simulink model "mind"  (R2022b)
settings: Solver=FixedStepAuto  StartTime=0.0  StopTime=inf  RelTol=1e-3  EnableMultiTasking=on
undefined symbols (not defined in the file or in its folder): DiscIntNeverNeededParam, GRM_discrete, HinfDiscrete, K, Observer, PID, Red
libraries: arduinolib x5, simulink x1, slpidlib x1
settings Model: SimulationMode=external  ExtModeTrigDuration=2  Creator=amoralesma  LastModifiedBy=amoralesma
settings DataIOCC: ReturnWorkspaceOutputs=off
settings OptimizationCC: EnhancedBackFolding=on  PassReuseOutputArgsAs=Individual arguments  ZeroExternalMemoryAtStartup=off  ZeroInternalMemoryAtStartup=off  MaxStackSize=64  OptimizeBlockOrder=speed  DifferentSizesBufferReuse=on  OptimizationCustomize=off  EfficientTunableParamExpr=on
settings DebuggingCC: ParameterTunabilityLossMsg=error
settings HardwareCC: ProdBitPerInt=16  ProdBitPerPointer=16  ProdBitPerSizeT=16  ProdBitPerPtrDiffT=16  ProdLargestAtomicFloat=None  ProdWordSize=8  ProdHWDeviceType=Atmel->AVR  UseEmbeddedCoderFeatures=off  UseSimulinkCoderFeatures=off
settings SFSimCC: MATLABDynamicMemAlloc=off
settings RTWCC: Description=Embedded Coder  SystemTargetFile=ert.tlc  HardwareBoard=Arduino Mega 2560  TemplateMakefile=ert_default_tmf  RTWVerbose=off  Toolchain=Arduino AVR  BuildConfiguration=Faster Runs
settings CodeAppCC: ForceParamTrailComments=on  OperatorAnnotations=on  SimulinkDataObjDesc=on  SFDataObjDesc=on  MangleLength=10  InsertBlockDesc=on
settings ERTTargetCC: SupportContinuousTime=on  SupportNonInlinedSFcns=on  SupportVariableSizeSignals=on  ExtMode=on  ExtModeTransport=3  ExtModeStaticAlloc=on  ExtModeAutomaticAllocSize=off  ExtModeStaticAllocSize=2048  ExtModeMexFile=ext_xcp  ExtModeMexArgs=0 '/dev/cu.usbserial-14110' 115200  ExtModeIntrfLevel=Level2 - Open  ERTSrcFileBannerTemplate=codertarget_code_template.cgt  ERTHdrFileBannerTemplate=codertarget_code_template.cgt  ERTDataSrcFileTemplate=codertarget_code_template.cgt  ERTDataHdrFileTemplate=codertarget_code_template.cgt

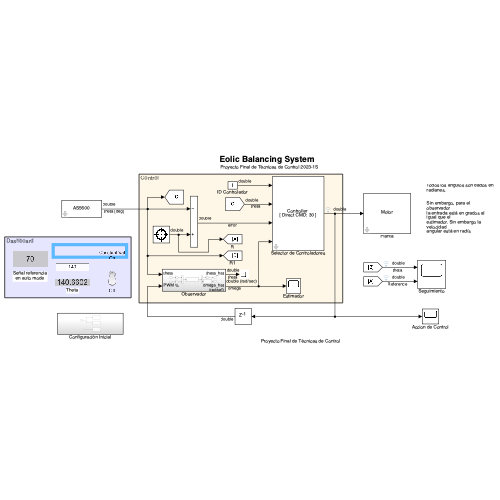
[thumbnail: Simulink's stored preview of the top-level diagram]
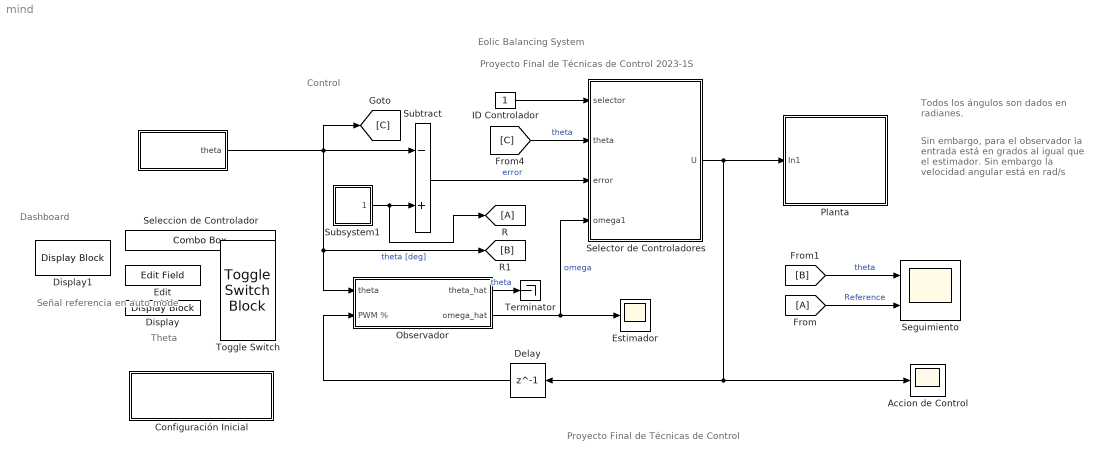
== system mind ==
  note: Señal referencia
      | en auto mode
  note: Dashboard
  note: Todos los ángulos son dados en
      | radianes.
  note: Control
  note: Eolic Balancing System
  note: Proyecto Final de Técnicas de Control 2023-1S
  note: Sin embargo, para el observador
      | la entrada está en grados al igual que el
      | estimador. Sin embargo la velocidad
      | angular está en rad/s
  note: Proyecto Final de Técnicas de Control
  note: Theta
  " " : Subsystem
      mask Display: disp('AS5600');
  Accion de Control : Scope
  Configuración Inicial : Subsystem
  Delay : Delay  DelayLength=1
  Display : DisplayBlock  LabelPosition=Hide  Transparency=1
  Display1 : DisplayBlock  LabelPosition=Hide  Transparency=1
  Edit : EditField  LabelPosition=Hide  ShowInitialText=on  Alignment=Center
  Estimador : Scope
  From : From
  ID Controlador : Constant  SampleTime=0.0025
  Observador : Subsystem
  Planta : Subsystem
      mask Display: disp('Motor');
  R : Goto
  Seguimiento : Scope  NumInputPorts=2
  Seleccion de Controlador : ComboBox  LabelPosition=Hide  SelectedLabel=PID + Red
      settings: Values={{'PID + Red', 'SMC', 'H-infinito', 'SMC + tanh', 'SMC + equivalente', 'MRAC', 'LQR', 'LQG'}, [1 2 3 4 5 6 7 8]}
  Selector de Controladores : Subsystem  mask{accionControlDirecta=30}
      mask prompts: accionControlDirecta "Accion de Control Directa"
      mask DialogControl DescTextVar Prompt: Selector de controladores. Varía el controlador en función del a entrada ID
      mask Display: disp("Controller \n[ Direct CMD: " + get_param(gcb, "accionControlDirecta") + " ]");
  Subsystem1 : Subsystem
      mask Display: image('/Users/amoralesma/Documents/UN/TdC/eolic-balancing-cs/implementacion/assets/target_icon.png'); % Use "Edit Image" on toolstrip to change.
  Subtract : Sum  Inputs=-+
  Terminator : Terminator
  Toggle Switch : ToggleSwitchBlock
      settings: Values={{'Off', 'On'}, [0 1]}
  wires:
  " "/1(theta) -> [C], Subtract/1, [B], Observador/1(theta)  "theta [deg]"
  Subtract/1 -> Selector de Controladores/3(error)  "error"
  Selector de Controladores/1(U) -> Delay/1, Accion de Control/1, Planta/1(In1)
  ID Controlador/1 -> Selector de Controladores/1(selector)
  Observador/2(omega_hat) -> Selector de Controladores/4(omega1), Estimador/1  "omega"
  Delay/1 -> Observador/2(PWM %)
  From/1 -> Seguimiento/2  "Reference"
  [B] -> Seguimiento/1  "theta"
  Observador/1(theta_hat) -> Terminator/1  "theta"
  [C] -> Selector de Controladores/2(theta)  "theta"
  Subsystem1/1(Out2) -> R/1, Subtract/2

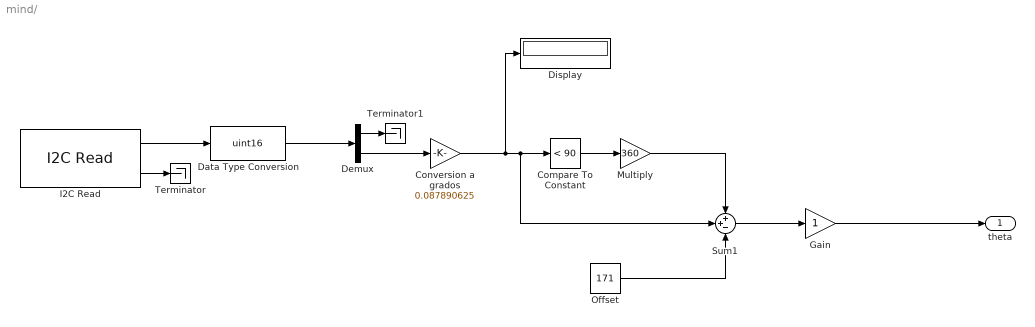
== system mind/  ==
  Compare To Constant : simulink/Logic and Bit Operations/Compare To Constant  relop=<  const=90  OutDataTypeStr=uint8
  Conversion a grados : Gain  Gain=0.087890625
  Data Type Conversion : DataTypeConversion  OutDataTypeStr=uint16  SaturateOnIntegerOverflow=off  RndMeth=Floor
  Demux : Demux  Outputs=2
  Display : Display
  Gain : Gain
  I2C Read : arduinolib/I2C Read  I2CModule=0  Mode=Master  SlaveAddress=0x36  SlaveByteOrder=BigEndian  Direction=Receiver  RegisterAddressMode=on  RegisterAddress=0x0C  SlaveDataType=uint16  DataLength=2  NoAck=off  RepeatedStart=off  OutputStatus=on  blockPlatform=ARDUINO  SampleTime=-1
  Multiply : Gain  Gain=360
  Offset : Constant  Value=171
  Sum1 : Sum  Inputs=++-
  Terminator : Terminator
  Terminator1 : Terminator
  theta : Outport
  wires:
  Demux/2 -> Conversion a grados/1
  Data Type Conversion/1 -> Demux/1
  Offset/1 -> Sum1/3
  I2C Read/1 -> Data Type Conversion/1
  Multiply/1 -> Sum1/1
  Conversion a grados/1 -> Display/1, Compare To Constant/1, Sum1/2
  Compare To Constant/1 -> Multiply/1
  I2C Read/2 -> Terminator/1
  Sum1/1 -> Gain/1
  Demux/1 -> Terminator1/1
  Gain/1 -> theta/1

== system mind/Configuración Inicial ==
  Constant : Constant
  Constant1 : Constant  Value=0
  EN1 : arduinolib/Digital Output  pinNumber=11  Direction=output  blockPlatform=arduino
  EN2 : arduinolib/Digital Output  pinNumber=12  Direction=output  blockPlatform=arduino
  IN3 : arduinolib/Digital Output  pinNumber=6  Direction=output  blockPlatform=arduino
  wires:
  Constant/1 -> EN2/1, EN1/1
  Constant1/1 -> IN3/1

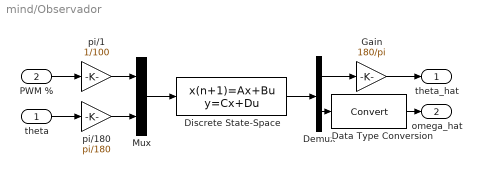
== system mind/Observador ==
  theta : Inport
  PWM % : Inport  Port=2
  Data Type Conversion : DataTypeConversion  SaturateOnIntegerOverflow=off  RndMeth=Floor
  Demux : Demux  Outputs=2
  Discrete State-Space : DiscreteStateSpace  A=Observer.A  B=Observer.B  C=Observer.C  D=Observer.D  SampleTime=-1
  Gain : Gain  Gain=180/pi
  Mux : Mux  Inputs=2
  pi/1 : Gain  Gain=1/100  OutDataTypeStr=Inherit: Same as input
  pi/180 : Gain  Gain=pi/180
  theta_hat : Outport
  omega_hat : Outport  Port=2  Unit=rad/sec
  wires:
  Mux/1 -> Discrete State-Space/1
  theta/1 -> pi/180/1
  Discrete State-Space/1 -> Demux/1
  pi/180/1 -> Mux/2
  PWM %/1 -> pi/1/1
  pi/1/1 -> Mux/1
  Gain/1 -> theta_hat/1
  Demux/1 -> Gain/1
  Demux/2 -> Data Type Conversion/1
  Data Type Conversion/1 -> omega_hat/1

== system mind/Planta ==
  In1 : Inport
  Gain1 : Gain  Gain=255/100
  PWM : arduinolib/PWM  pinNumber=7  frequencyType=Default  desiredFrequency=490.2  achievableFrequency=490.2
  wires:
  In1/1 -> Gain1/1
  Gain1/1 -> PWM/1

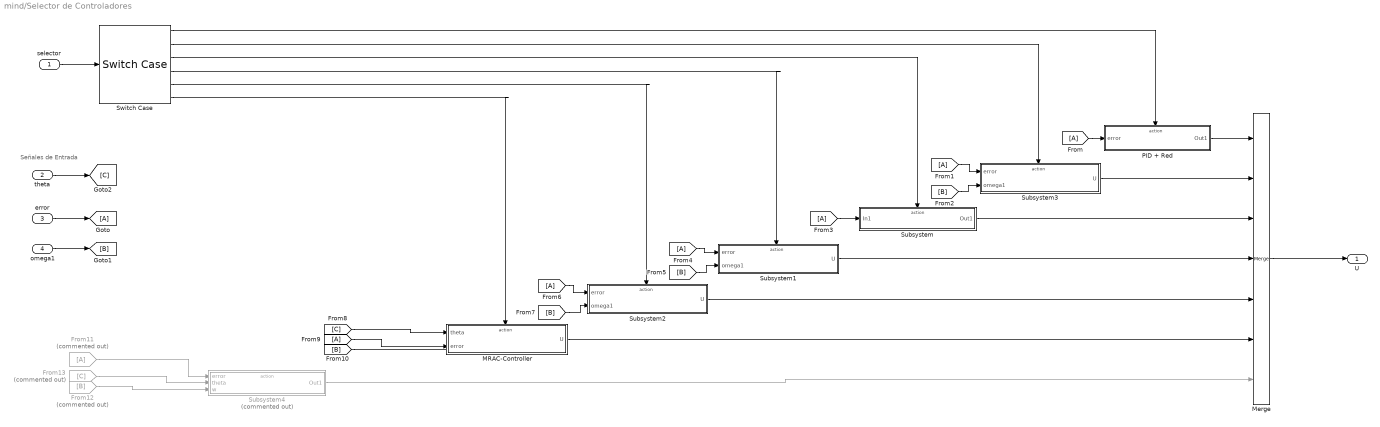
== system mind/Selector de Controladores ==
  note: Señales de Entrada
  selector : Inport
  theta : Inport  Port=2
  error : Inport  Port=3
  omega1 : Inport  Port=4
  From{,1,3..4,6,9} (6 alike) : From
  From11 : From  Commented=on
  From12 : From  Commented=on  GotoTag=B
  From13 : From  Commented=on  GotoTag=C
  Goto : Goto
  MRAC-Controller : Subsystem  mask{directCMD=accionControlDirecta, gx=7, gr=0.3}
      mask prompts: directCMD "CMD"; gx "Gamma X"; gr "Gamma R"
      mask DialogControl Control2 Prompt: Propiedades de MRAC
      mask Display:
      | disp('MRAC');
      | 
      | port_label('input', 1, 'theta');
      | port_label('input', 2, 'error');
      | port_label('input', 3, 'omega');
      | 
      | port_label('output', 1, 'u');
  Merge : Merge  Inputs=7
  PID + Red : Subsystem  mask{directCMD=accionControlDirecta}
      mask prompts: directCMD "Accion de control directa"
      mask Display: disp('PID');
  Subsystem : Subsystem
      mask Display: disp('H-inf');
  Subsystem1 : Subsystem
      mask Display:
      | disp('SMC + tanh');
      | 
      | port_label('input', 1, 'error');
      | port_label('input', 2, 'omega (x2)');
      | 
      | port_label('output', 1, 'u');
  Subsystem2 : Subsystem
      mask Display:
      | disp('SMC + eq');
      | 
      | port_label('input', 1, 'error');
      | port_label('input', 2, 'omega (x2)');
      | 
      | port_label('output', 1, 'u');
  Subsystem3 : Subsystem
      mask Display:
      | disp('SMC');
      | 
      | port_label('input', 1, 'error');
      | port_label('input', 2, 'omega (x2)');
      | 
      | port_label('output', 1, 'u');
  Subsystem4 : Subsystem  Commented=on
      mask Display: disp('LQR');
  Switch Case : SwitchCase  CaseConditions={1, 2,3, 4, 5,6,}  ShowDefaultCase=off
  U : Outport
  wires:
  Switch Case/1 -> PID + Red/Action
  Switch Case/2 -> Subsystem3/Action
  error/1 -> Goto/1
  omega1/1 -> [B]
  From/1 -> PID + Red/1(error)
  From1/1 -> Subsystem3/1(error)
  [B] -> Subsystem3/2(omega1)
  PID + Red/1(Out1) -> Merge/1
  Subsystem3/1(U) -> Merge/2
  selector/1 -> Switch Case/1
  From3/1 -> Subsystem/1(In1)
  Subsystem/1(Out1) -> Merge/3
  Switch Case/3 -> Subsystem/Action
  Merge/1 -> U/1
  Switch Case/4 -> Subsystem1/Action
  Switch Case/5 -> Subsystem2/Action
  From4/1 -> Subsystem1/1(error)
  [B] -> Subsystem1/2(omega1)
  From6/1 -> Subsystem2/1(error)
  [B] -> Subsystem2/2(omega1)
  Subsystem1/1(U) -> Merge/4
  Subsystem2/1(U) -> Merge/5
  Switch Case/6 -> MRAC-Controller/Action
  theta/1 -> [C]
  [C] -> MRAC-Controller/1(theta)
  From9/1 -> MRAC-Controller/2(error)
  MRAC-Controller/1(U) -> Merge/6
  [B] -> ?
  Subsystem4/1(Out1) -> Merge/7
  From13/1 -> Subsystem4/2(theta)
  From12/1 -> Subsystem4/3(w)
  From11/1 -> Subsystem4/1(error)

== system mind/Subsystem1 ==
  Constant : Constant  Value=0
  Ref : Constant  Value=140
  Subsystem : Subsystem
  Switch : Switch  Criteria=u2 ~= 0  SaturateOnIntegerOverflow=off  InputSameDT=off
  Out2 : Outport
  wires:
  Switch/1 -> Out2/1
  Constant/1 -> Switch/2
  Subsystem/1(Out1) -> Switch/1
  Ref/1 -> Switch/3

== system mind/Selector de Controladores/MRAC-Controller ==
  theta : Inport
  error : Inport  Port=2
  Action Port : ActionPort  ActionPortLabel=case [ 6 ]:
  Gain : Gain  Gain=pi/180
  Gain1 : Gain  Gain=pi/180
  MRAC : Subsystem
  U : Outport
  wires:
  theta/1 -> Gain/1
  error/1 -> Gain1/1
  Gain1/1 -> MRAC/2(error)
  MRAC/1(U) -> U/1
  Gain/1 -> MRAC/1(theta)

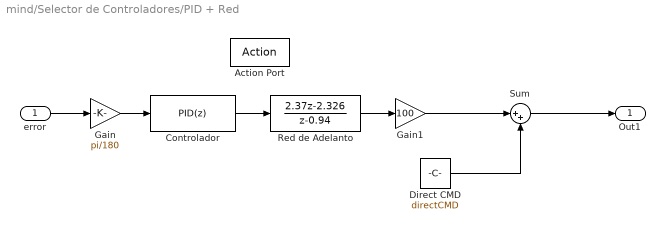
== system mind/Selector de Controladores/PID + Red ==
  error : Inport
  Action Port : ActionPort  ActionPortLabel=case [ 1 ]:
  Controlador : slpidlib/PID Controller  Controller=PID  Form=Parallel  TimeDomain=Discrete-time  UseExternalTs=off  SampleTime=0.0025  IntegratorMethod=Forward Euler  FilterMethod=Forward Euler  ControllerParametersSource=internal  P=0.4  I=0.65  UseKiTs=off  D=0.018  N=100  UseFilter=off  TunerSelectOption=Transfer Function Based (PID Tuner App)  InitialConditionSource=internal  InitialConditionForIntegrator=0  InitialConditionForFilter=0  DifferentiatorICPrevScaledInput=0  ExternalReset=none  TrackingMode=off  Kt=1  LimitOutput=on  SatLimitsSource=internal  UpperSaturationLimit=70  LowerSaturationLimit=-30  LinearizeAsGain=off  AntiWindupMode=clamping  Kb=1.1  LimitIntegrator=on  UpperIntegratorSaturationLimit=70  LowerIntegratorSaturationLimit=-30  POutMin=[]  POutMax=[]  IOutMin=[]  IOutMax=[]  DOutMin=[]  DOutMax=[]  NOutMin=[]  NOutMax=[]  SumOutMin=[]  SumOutMax=[]  SaturationOutMin=[]  SaturationOutMax=[]  PParamMin=[]  PParamMax=[]  IParamMin=[]  IParamMax=[]  DParamMin=[]  DParamMax=[]  NParamMin=[]  NParamMax=[]  KbParamMin=[]  KbParamMax=[]  KtParamMin=[]  KtParamMax=[]  KbOutMin=[]  KbOutMax=[]  KtOutMin=[]  KtOutMax=[]  IntegratorOutMin=[]  IntegratorOutMax=[]  FilterOutMin=[]  FilterOutMax=[]  SumI1OutMin=[]  SumI1OutMax=[]  SumI2OutMin=[]  SumI2OutMax=[]  SumI3OutMin=[]  SumI3OutMax=[]  SumI4OutMin=[]  SumI4OutMax=[]  SumDOutMin=[]  SumDOutMax=[]  DifferentiatorOutMin=[]  DifferentiatorOutMax=[]  FilterDiffOutCoefMin=[]  FilterDiffOutCoefMax=[]  ReciprocalOutMin=[]  ReciprocalOutMax=[]  SumDenOutMin=[]  SumDenOutMax=[]  SumNumOutMin=[]  SumNumOutMax=[]  DivideOutMin=[]  DivideOutMax=[]  UdiffTsProdOutMin=[]  UdiffTsProdOutMax=[]  NTsProdOutMin=[]  NTsProdOutMax=[]  UintegralTsProdOutMin=[]  UintegralTsProdOutMax=[]  UngainTsProdOutMin=[]  UngainTsProdOutMax=[]  ClampingZeroOutDataTypeStr=Inherit: Inherit via back propagation  ClampingZeroOutMin=[]  ClampingZeroOutMax=[]  FilterDenConstantOutDataTypeStr=Inherit: Inherit via back propagation  FilterDenConstantOutMin=[]  FilterDenConstantOutMax=[]  PCopyOutDataTypeStr=Inherit: Inherit via back propagation  PCopyOutMin=[]  PCopyOutMax=[]  NCopyOutDataTypeStr=Inherit: Inherit via back propagation  NCopyOutMin=[]  NCopyOutMax=[]  IntegratorContinuousStateAttributes=''  IntegratorStateMustResolveToSignalObject=off  IntegratorRTWStateStorageClass=Auto  FilterContinuousStateAttributes=''  FilterStateMustResolveToSignalObject=off  FilterRTWStateStorageClass=Auto  ParallelPVariant=InternalParameters  IdealPVariant=Disabled  IVariant=InternalParameters  DVariant=InternalParameters  IntegratorVariant=Discrete  SatVariant=Enabled  AWVariant=DiscClampingParallel  PCopyVariant=Disabled  TRVariant=Disabled  FdbkBlocksVariant=Forward  IdealPFdbkVariant=Disabled  SatFdbkVariant=Disabled  DerivativeFilterVariant=Differentiator  NVariant=Passthrough  NCopyVariant=Disabled_SignalSpec  FilterICVariant=InternalICsDifferentiator  IntegratorICVariant=InternalICs  ExternalResetVariant=Disabled  TRSumVariant=Passthrough  SumFdbkVariant=Disabled  SumVariant=Sum_PID  TsampFilterVariant=InternalTs  TsampNgainVariant=Passthrough  TsampIntegralVariant=Passthrough  ExternalSaturationOutDataTypeStr=Inherit: Same as second input
      settings: LibrarySourceBlock=simulink/Discrete/Discrete PID Controller
  Direct CMD : Constant  Value=directCMD
  Gain : Gain  Gain=pi/180
  Gain1 : Gain  Gain=100
  Red de Adelanto : DiscreteTransferFcn  Numerator=[2.37 -2.326]  Denominator=[1 -0.94]
  Sum : Sum  Inputs=|++
  Out1 : Outport
  wires:
  error/1 -> Gain/1
  Red de Adelanto/1 -> Gain1/1
  Gain/1 -> Controlador/1
  Controlador/1 -> Red de Adelanto/1
  Sum/1 -> Out1/1
  Gain1/1 -> Sum/1
  Direct CMD/1 -> Sum/2

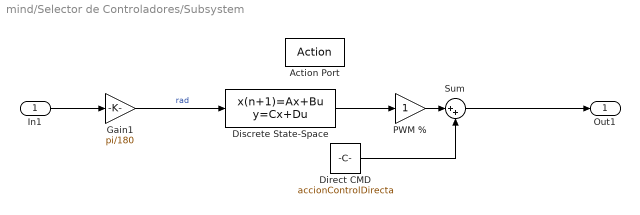
== system mind/Selector de Controladores/Subsystem ==
  In1 : Inport
  Action Port : ActionPort  ActionPortLabel=case [ 3 ]:
  Direct CMD : Constant  Value=accionControlDirecta
  Discrete State-Space : DiscreteStateSpace  A=HinfDiscrete.A  B=HinfDiscrete.B  C=HinfDiscrete.C  D=HinfDiscrete.D  SampleTime=-1
  Gain1 : Gain  Gain=pi/180
  PWM % : Gain
  Sum : Sum  Inputs=|++
  Out1 : Outport
  wires:
  Discrete State-Space/1 -> PWM %/1
  In1/1 -> Gain1/1
  Gain1/1 -> Discrete State-Space/1  "rad"
  Direct CMD/1 -> Sum/2
  PWM %/1 -> Sum/1
  Sum/1 -> Out1/1

== system mind/Selector de Controladores/Subsystem1 ==
  error : Inport
  omega1 : Inport  Port=2
  Action Port : ActionPort  ActionPortLabel=case [ 4 ]:
  Delay : Delay  DelayLength=1
  Gain : Gain  Gain=pi/180
  Saturation : Saturate  UpperLimit=80  LowerLimit=10
  Subsystem2 : Subsystem
  U : Outport
  wires:
  omega1/1 -> Subsystem2/2(omega1)
  error/1 -> Gain/1
  Subsystem2/1(U) -> Delay/1
  Gain/1 -> Subsystem2/1(error)
  Delay/1 -> Saturation/1
  Saturation/1 -> U/1

== system mind/Selector de Controladores/Subsystem2 ==
  error : Inport
  omega1 : Inport  Port=2
  Action Port : ActionPort  ActionPortLabel=case [ 5 ]:
  Delay : Delay  DelayLength=1
  Gain : Gain  Gain=pi/180
  Saturation : Saturate  UpperLimit=80  LowerLimit=10
  Subsystem2 : Subsystem
  U : Outport
  wires:
  omega1/1 -> Subsystem2/2(omega1)
  error/1 -> Gain/1
  Subsystem2/1(U) -> Delay/1
  Gain/1 -> Subsystem2/1(error)
  Delay/1 -> Saturation/1
  Saturation/1 -> U/1

== system mind/Selector de Controladores/Subsystem3 ==
  error : Inport
  omega1 : Inport  Port=2
  Action Port : ActionPort  ActionPortLabel=case [ 2 ]:
  Delay : Delay  DelayLength=1
  Gain : Gain  Gain=pi/180
  Saturation : Saturate  UpperLimit=80  LowerLimit=10
  Subsystem2 : Subsystem
  U : Outport
  wires:
  omega1/1 -> Subsystem2/2(omega1)
  error/1 -> Gain/1
  Subsystem2/1(U) -> Delay/1
  Gain/1 -> Subsystem2/1(error)
  Delay/1 -> Saturation/1
  Saturation/1 -> U/1

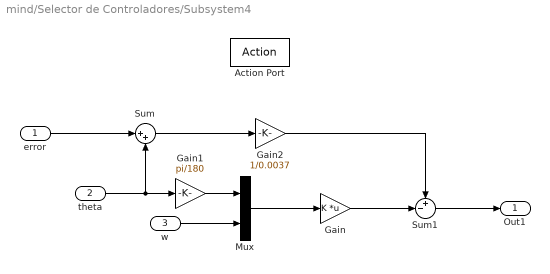
== system mind/Selector de Controladores/Subsystem4 ==
  error : Inport
  theta : Inport  Port=2
  w : Inport  Port=3
  Action Port : ActionPort
  Gain : Gain  Gain=K  Multiplication=Matrix(K*u)
  Gain1 : Gain  Gain=pi/180
  Gain2 : Gain  Gain=1/0.0037
  Mux : Mux  Inputs=2
  Sum : Sum  Inputs=|++
  Sum1 : Sum  Inputs=+-|
  Out1 : Outport
  wires:
  w/1 -> Mux/2
  Mux/1 -> Gain/1
  Gain1/1 -> Mux/1
  theta/1 -> Sum/2, Gain1/1
  error/1 -> Sum/1
  Sum/1 -> Gain2/1
  Gain/1 -> Sum1/2
  Sum1/1 -> Out1/1
  Gain2/1 -> Sum1/1

== system mind/Subsystem1/Subsystem ==
  Step : Step  Time=20  Before=70  After=90  SampleTime=0
  Step1 : Step  Time=40  After=-30  SampleTime=0
  Step2 : Step  Time=60  After=10  SampleTime=0
  Sum : Sum  Inputs=+++
  Out1 : Outport
  wires:
  Step/1 -> Sum/1
  Step2/1 -> Sum/3
  Step1/1 -> Sum/2
  Sum/1 -> Out1/1

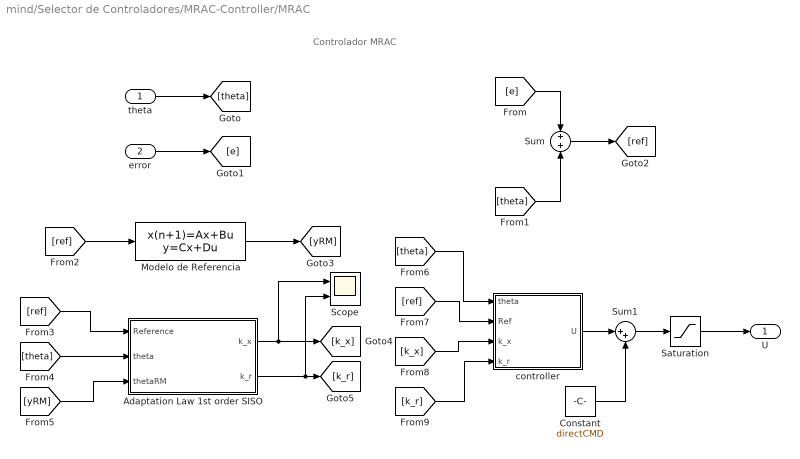
== system mind/Selector de Controladores/MRAC-Controller/MRAC ==
  note: Controlador MRAC
  theta : Inport
  error : Inport  Port=2
  Adaptation Law 1st order SISO : Subsystem
  Constant : Constant  Value=directCMD
  Modelo de Referencia : DiscreteStateSpace  A=GRM_discrete.A  B=GRM_discrete.B  C=GRM_discrete.C  D=GRM_discrete.D  SampleTime=2.5e-3
  Saturation : Saturate  UpperLimit=100  LowerLimit=0
  Scope : Scope  NumInputPorts=2
  Sum : Sum
  Sum1 : Sum  Inputs=|++
  controller : Subsystem
  U : Outport
  wires:
  theta/1 -> [theta]
  error/1 -> [e]
  [e] -> Sum/1
  [theta] -> Sum/2
  Sum/1 -> [ref]
  [ref] -> Modelo de Referencia/1
  Modelo de Referencia/1 -> [yRM]
  [ref] -> Adaptation Law 1st order SISO/1(Reference)
  [theta] -> Adaptation Law 1st order SISO/2(theta)
  [yRM] -> Adaptation Law 1st order SISO/3(thetaRM)
  Adaptation Law 1st order SISO/1(k_x) -> Scope/1, [k_x]
  Adaptation Law 1st order SISO/2(k_r) -> Scope/2, [k_r]
  Saturation/1 -> U/1
  [theta] -> controller/1(theta)
  [ref] -> controller/2(Ref)
  [k_r] -> controller/4(k_r)
  [k_x] -> controller/3(k_x)
  Sum1/1 -> Saturation/1
  controller/1(U) -> Sum1/1
  Constant/1 -> Sum1/2

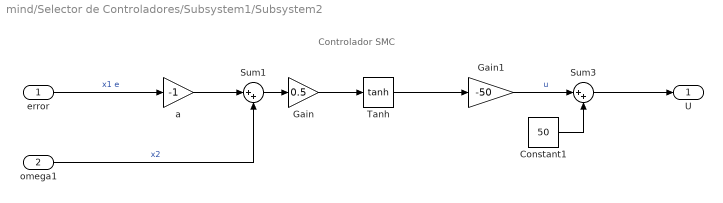
== system mind/Selector de Controladores/Subsystem1/Subsystem2 ==
  note: Controlador SMC
  error : Inport
  omega1 : Inport  Port=2
  Constant1 : Constant  Value=50
  Gain : Gain  Gain=0.5
  Gain1 : Gain  Gain=-50
  Sum1 : Sum  Inputs=|++
  Sum3 : Sum  Inputs=|++
  Tanh : Trigonometry  Operator=tanh
  a : Gain  Gain=-1
  U : Outport
  wires:
  a/1 -> Sum1/1
  omega1/1 -> Sum1/2  "x2"
  error/1 -> a/1  "x1 e"
  Gain1/1 -> Sum3/1  "u"
  Constant1/1 -> Sum3/2
  Sum1/1 -> Gain/1
  Sum3/1 -> U/1
  Tanh/1 -> Gain1/1
  Gain/1 -> Tanh/1

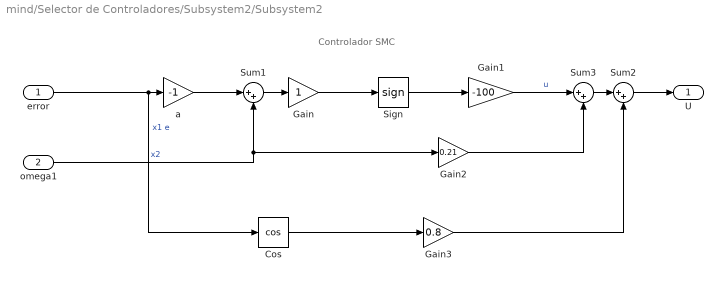
== system mind/Selector de Controladores/Subsystem2/Subsystem2 ==
  note: Controlador SMC
  error : Inport
  omega1 : Inport  Port=2
  Cos : Trigonometry  Operator=cos
  Gain : Gain
  Gain1 : Gain  Gain=-100
  Gain2 : Gain  Gain=0.21
  Gain3 : Gain  Gain=0.8
  Sign : Signum
  Sum1 : Sum  Inputs=|++
  Sum2 : Sum  Inputs=|++
  Sum3 : Sum  Inputs=|++
  a : Gain  Gain=-1
  U : Outport
  wires:
  a/1 -> Sum1/1
  omega1/1 -> Sum1/2, Gain2/1  "x2"
  error/1 -> Cos/1, a/1  "x1 e"
  Gain1/1 -> Sum3/1  "u"
  Sum1/1 -> Gain/1
  Sign/1 -> Gain1/1
  Gain/1 -> Sign/1
  Sum3/1 -> Sum2/1
  Sum2/1 -> U/1
  Gain2/1 -> Sum3/2
  Cos/1 -> Gain3/1
  Gain3/1 -> Sum2/2

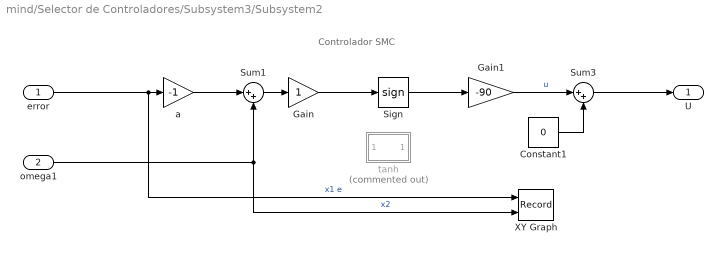
== system mind/Selector de Controladores/Subsystem3/Subsystem2 ==
  note: Controlador SMC
  error : Inport
  omega1 : Inport  Port=2
  Constant1 : Constant  Value=0
  Gain : Gain
  Gain1 : Gain  Gain=-90
  Sign : Signum
  Sum1 : Sum  Inputs=|++
  Sum3 : Sum  Inputs=|++
  XY Graph : Record  FileSettingsInternal="{\"entries\":[{\"content\":{\"excelSettings\":{\"content\":{},\"type\":\"Streamout.ExcelSettings\"}},\"type\":\"Streamout.FileSettingStorage\",\"uuid\":\"357fd5d7-b37b-410e-bb48-35e93cbaef29\"}],\"packageUris\":[\"http://schema.mathworks.com/mf0/streamout_blocks/R2020a\"],\"version\":\"1.0\"}"  Layout=[1 1]  SignalsInternal="{\"entries\":[{\"content\":{\"signals\":[{\"content\":{\"blockPath\":[\"mind/Selector de Controladores/Subsystem3/Subsystem2/XY Graph\"],\"channel\":[],\"dimensions\":[1,1],\"domain\":\"mind/Selector de Controladores/Subsystem3/Subsystem2/XY Graph\",\"lineColor\":\"#a2142f\",\"plots\":[1],\"port\":1,\"sid\":[\"617\"],\"signalID\":602268,\"signalName\":\"x1 e\"},\"type\":\"RecordBlkView.Signal\",\"uuid\":\"f3fd6ff8-eec6-438a-af7c-cbc8a6a581d5\"},{\"content\":{\"blockPath\":[\"mind/Selector de Controladores/Subsystem3/Subsystem2/XY Graph\"],\"channel\":[],\"dimensions\":[1],\"domain\":\"mind/Selector de Controladores/Subsystem3/Subsystem2/XY Graph\",\"lineColor\":\"#139fff\",\"plots\":[1],\"port\":2,\"sid\":[\"617\"],\"signalID\":602272,\"signalName\":\"x2\"},\"type\":\"RecordBlkView.Signal\",\"uuid\":\"ca2baead-f382-4316-9b22-44514c630c3b\"}]},\"type\":\"RecordBlkView.InputSignals\",\"uuid\":\"79c0466b-0b60-4e59-8ebb-c374b083f65a\"}],\"packageUris\":[\"http://schema.mathworks.com/mf0/streamout_blocks/R2020a\"],\"version\":\"1.0\"}"  VisualizationBindings="{\"xyplotplugin\":{\"info\":[{\"series\":[{\"bindingParametersList\":[{\"parameter\":\"X-Axis\",\"signalID\":602268,\"signalName\":\"x1 e\"},{\"parameter\":\"Y-Axis\",\"signalID\":602272,\"signalName\":\"x2\"}],\"seriesID\":19952}],\"subplotID\":1}]}}"  CompatibilityTag=XY
  a : Gain  Gain=-1
  tanh : Subsystem  Commented=on
  U : Outport
  wires:
  a/1 -> Sum1/1
  omega1/1 -> XY Graph/2, Sum1/2  "x2"
  error/1 -> XY Graph/1, a/1  "x1 e"
  Gain1/1 -> Sum3/1  "u"
  Constant1/1 -> Sum3/2
  Sum1/1 -> Gain/1
  Sum3/1 -> U/1
  Sign/1 -> Gain1/1
  Gain/1 -> Sign/1

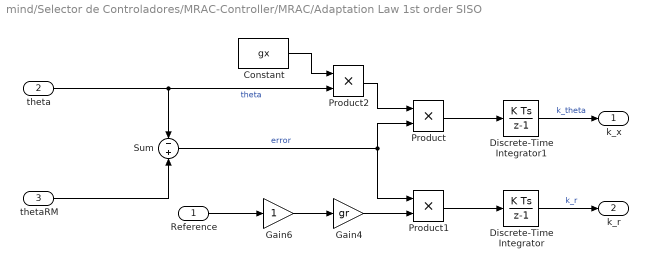
== system mind/Selector de Controladores/MRAC-Controller/MRAC/Adaptation Law 1st order SISO ==
  Reference : Inport
  theta : Inport  Port=2
  thetaRM : Inport  Port=3
  Constant : Constant  Value=gx
  Discrete-Time Integrator : DiscreteIntegrator  SampleTime=2.5e-3  ICPrevOutput=DiscIntNeverNeededParam  ICPrevScaledInput=DiscIntNeverNeededParam
  Discrete-Time Integrator1 : DiscreteIntegrator  SampleTime=2.5e-3  ICPrevOutput=DiscIntNeverNeededParam  ICPrevScaledInput=DiscIntNeverNeededParam
  Gain4 : Gain  Gain=gr
  Gain6 : Gain
  Product : Product
  Product1 : Product
  Product2 : Product
  Sum : Sum  Inputs=-+
  k_x : Outport
  k_r : Outport  Port=2
  wires:
  Product1/1 -> Discrete-Time Integrator/1
  Reference/1 -> Gain6/1
  Sum/1 -> Product1/1, Product/2  "error"
  Gain6/1 -> Gain4/1
  Product2/1 -> Product/1
  Constant/1 -> Product2/1
  Discrete-Time Integrator/1 -> k_r/1  "k_r"
  Discrete-Time Integrator1/1 -> k_x/1  "k_theta"
  theta/1 -> Product2/2, Sum/1  "theta"
  thetaRM/1 -> Sum/2
  Gain4/1 -> Product1/2
  Product/1 -> Discrete-Time Integrator1/1

== system mind/Selector de Controladores/MRAC-Controller/MRAC/controller ==
  theta : Inport
  Ref : Inport  Port=2
  k_x : Inport  Port=3
  k_r : Inport  Port=4
  Product : Product
  Product2 : Product
  Sum : Sum
  U : Outport
  wires:
  Ref/1 -> Product/2
  Product/1 -> Sum/2
  k_r/1 -> Product/1
  k_x/1 -> Product2/1  "k_theta"
  Sum/1 -> U/1
  Product2/1 -> Sum/1
  theta/1 -> Product2/2

== system mind/Selector de Controladores/Subsystem3/Subsystem2/tanh ==
  In1 : Inport
  Tanh : Trigonometry  Operator=tanh  OutputSignalType=real
  Out1 : Outport
  wires:
  Tanh/1 -> Out1/1
  In1/1 -> Tanh/1
